simulink model "rossler"  (R2022b)
settings: Solver=VariableStepAuto  StartTime=0.0  StopTime=100  MaxStep=1e-4  RelTol=1e-3
settings Model: Creator=Dong  LastModifiedBy=Dong

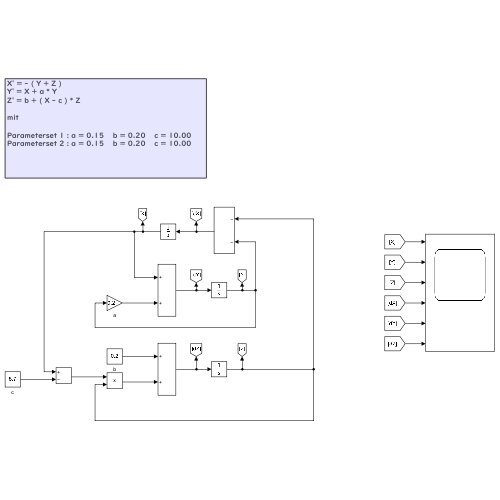
[thumbnail: Simulink's stored preview of the top-level diagram]
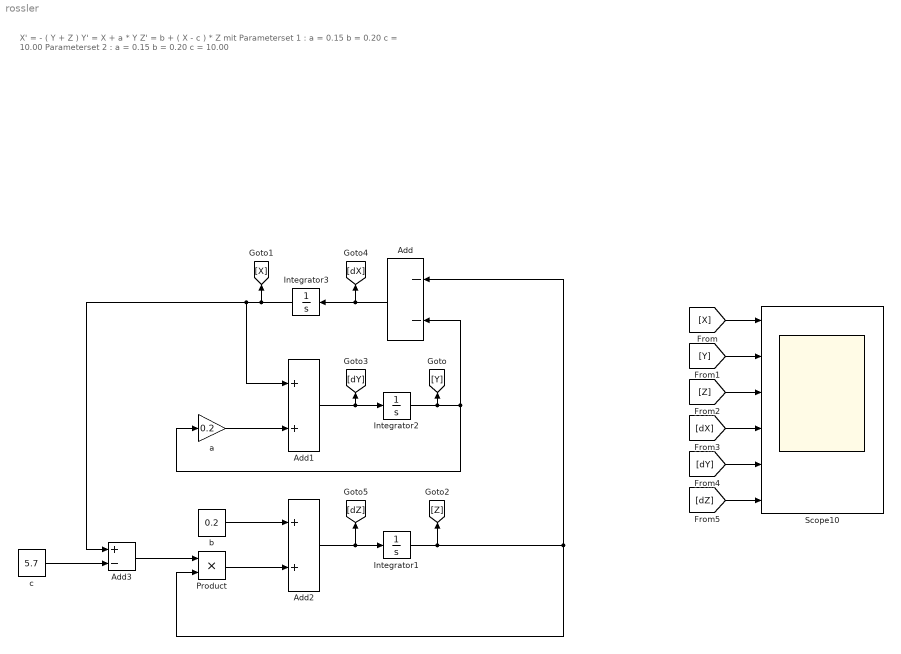
== system rossler ==
  note: X' = - ( Y + Z )
      | Y' = X + a * Y
      | Z' = b + ( X - c ) * Z
      |
      | mit
      |
      | Parameterset 1 : a = 0.15    b = 0.20    c = 10.00
      | Parameterset 2 : a = 0.15    b = 0.20    c = 10.00
  Add : Sum  Inputs=--
  Add1 : Sum
  Add2 : Sum
  Add3 : Sum  Inputs=+-
  Integrator1 : Integrator
  Integrator2 : Integrator
  Integrator3 : Integrator
  Product : Product
  Scope10 : Scope  NumInputPorts=6
  a : Gain  Gain=0.2
  b : Constant  Value=0.2
  c : Constant  Value=5.7
  wires:
  Add2/1 -> [dZ], Integrator1/1
  Add1/1 -> [dY], Integrator2/1
  a/1 -> Add1/2
  Integrator2/1 -> [Y], a/1, Add/2
  Integrator3/1 -> Add1/1, Add3/1, [X]
  b/1 -> Add2/1
  Product/1 -> Add2/2
  Integrator1/1 -> [Z], Product/2, Add/1
  Add3/1 -> Product/1
  c/1 -> Add3/2
  [dZ] -> Scope10/6
  [dY] -> Scope10/5
  [dX] -> Scope10/4
  [Z] -> Scope10/3
  [Y] -> Scope10/2
  [X] -> Scope10/1
  Add/1 -> Integrator3/1, [dX]
